simulink model "sampleModel2030"  (R2023a)
settings: Solver=VariableStepAuto  StartTime=0.0  StopTime=10.0  RelTol=1e-3
libraries: hdlsllib x4, simulink x2
settings Model: Creator=user1  LastModifiedBy=user1

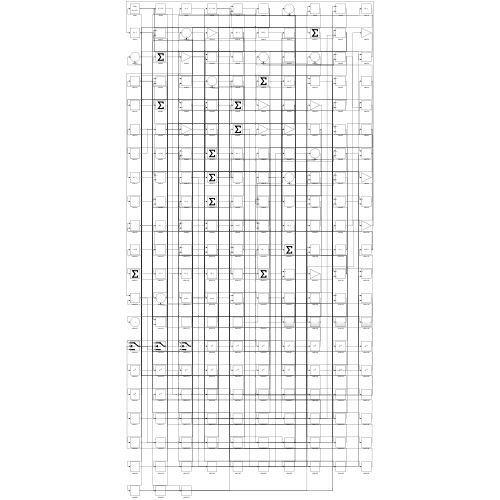
[thumbnail: Simulink's stored preview of the top-level diagram]
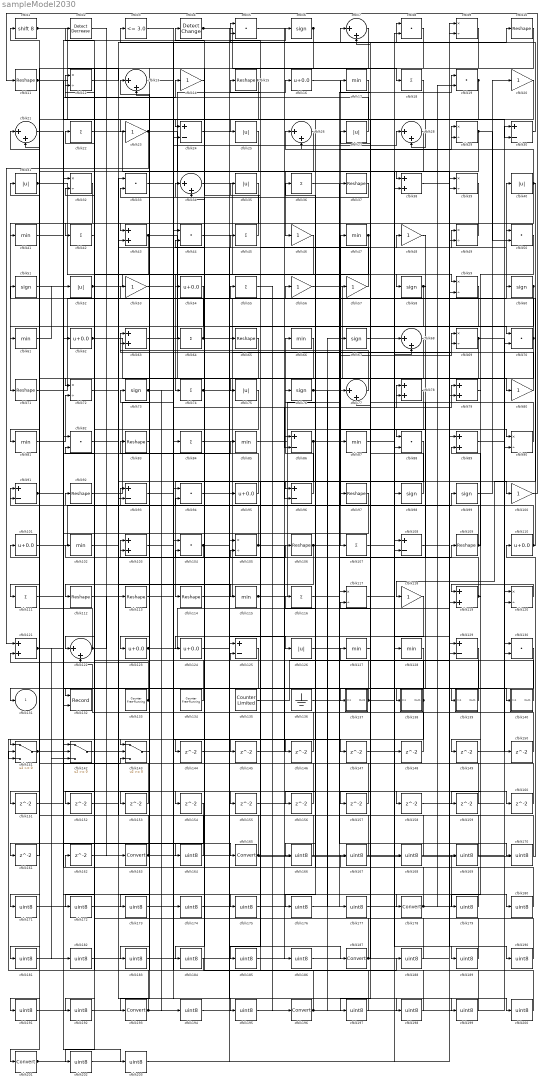
== system sampleModel2030 ==
  cfblk1 : ArithShift  BitShiftNumber=8
  cfblk{10..11,15,37,65,71,83,92,97,106,109,112..114} (14 alike) : Reshape
  cfblk{14,20,23,46,48,53,56..57,80,100,118} (11 alike) : Gain
  cfblk{16,54,62,95,101,110,123..124} (8 alike) : Bias  Bias=0.0  SaturateOnIntegerOverflow=off
  cfblk{17,41,47,61,66,81,85,87,102,115,127..128} (12 alike) : MinMax
  cfblk{38,43,63,78..79,89,103,119,121} (9 alike) : Sum
  cfblk{5,8,19,33,44,50,70,82,88,94,104,130} (12 alike) : DotProduct  OutDataTypeStr=Inherit: Inherit via internal rule
  cfblk{9,12,29,32,39,49,59,69,72,90,105,117,120} (13 alike) : Product  Inputs=*/  RndMeth=Zero  SaturateOnIntegerOverflow=on
  cfblk{18,22,36,42,45,55,64,74,84,107,111,116} (12 alike) : Sum  Inputs=+
  cfblk{24,30,86,91,93,96,108,125,129} (9 alike) : Sum  Inputs=+-
  cfblk{7,13,21,26,28,34,68,77,122} (9 alike) : Sum  Inputs=|++
  cfblk{25,27,31,35,40,52,75,126} (8 alike) : Abs  SaturateOnIntegerOverflow=off
  cfblk132 : Record  FileSettingsInternal="{\"entries\":[{\"content\":{\"excelSettings\":{\"content\":{},\"type\":\"Streamout.ExcelSettings\"}},\"type\":\"Streamout.FileSettingStorage\",\"uuid\":\"\"}],\"packageUris\":[\"http:\\/\\/schema.mathworks.com\\/mf0\\/streamout_blocks\\/R2020a\"],\"version\":\"1.0\"}"  Layout=[1 1]  SignalsInternal="{\"entries\":[{\"content\":{\"signals\":[{\"content\":{\"blockPath\":[],\"dimensions\":[1],\"domain\":\"\",\"lineColor\":\"#a2142f\",\"plots\":[1],\"port\":1,\"signalID\":6116,\"signalName\":\"XY Graph:1\"},\"type\":\"RecordBlkView.Signal\",\"uuid\":\"\"},{\"content\":{\"blockPath\":[],\"dimensions\":[1],\"domain\":\"\",\"lineColor\":\"#139fff\",\"plots\":[1],\"port\":2,\"signalID\":6119,\"signalName\":\"XY Graph:2\"},\"type\":\"RecordBlkView.Signal\",\"uuid\":\"\"}]},\"type\":\"RecordBlkView.InputSignals\",\"uuid\":\"\"}],\"packageUris\":[\"http:\\/\\/schema.mathworks.com\\/mf0\\/streamout_blocks\\/R2020a\"],\"version\":\"1.0\"}"  VisualizationBindings="{\"xyplotplugin\":{\"info\":[{\"series\":[{\"bindingParametersList\":[{\"parameter\":\"X-Axis\",\"signalID\":6116,\"signalName\":\"XY Graph:1\"},{\"parameter\":\"Y-Axis\",\"signalID\":6119,\"signalName\":\"XY Graph:2\"}],\"seriesID\":23883}],\"subplotID\":1}]}}"  CompatibilityTag=XY  st=-1
  cfblk133 : hdlsllib/Sources/Counter Free-Running  NumBits=16  tsamp=-1
  cfblk134 : hdlsllib/Sources/Counter Free-Running  NumBits=16  tsamp=-1
  cfblk135 : hdlsllib/Sources/Counter Limited  uplimit=7  tsamp=-1
  cfblk136 : Ground
  cfblk137 : Subsystem
      settings: LibrarySourceBlock=|
      | hdlsllib/Ports &
      | Subsystems/Subsystem
  cfblk138 : Subsystem
      settings: LibrarySourceBlock=|
      | hdlsllib/Ports &
      | Subsystems/Subsystem
  cfblk139 : Subsystem
      settings: LibrarySourceBlock=|
      | hdlsllib/Ports &
      | Subsystems/Subsystem
  cfblk140 : Subsystem
      settings: LibrarySourceBlock=|
      | hdlsllib/Ports &
      | Subsystems/Subsystem
  cfblk141 : Switch  SaturateOnIntegerOverflow=off  InputSameDT=off
  cfblk142 : Switch  SaturateOnIntegerOverflow=off  InputSameDT=off
  cfblk143 : Switch  SaturateOnIntegerOverflow=off  InputSameDT=off
  cfblk{144..162} (19 alike) : Delay  SampleTime=1
  cfblk{163,165,178,187,193,196,201} (7 alike) : DataTypeConversion  SaturateOnIntegerOverflow=off  RndMeth=Floor
  cfblk{164,166..177,179..186,188..192,194..195,197..200,202..203} (34 alike) : DataTypeConversion  OutDataTypeStr=uint8  SaturateOnIntegerOverflow=off  RndMeth=Floor
  cfblk2 : simulink/Logic and Bit Operations/Detect Decrease  vinit=0.0  OutDataTypeStr=boolean
      settings: LibrarySourceBlock=|
      | hdlsllib/Logic and Bit
      | Operations/Detect
      | Decrease
  cfblk3 : hdlsllib/Logic and Bit Operations/Compare To Constant  relop=<=  const=3.0  OutDataTypeStr=boolean
  cfblk4 : simulink/Logic and Bit Operations/Detect Change  vinit=0  OutDataTypeStr=boolean
      settings: LibrarySourceBlock=|
      | hdlsllib/Logic and Bit
      | Operations/Detect
      | Change
  cfblk{6,51,58,60,67,73,76,98..99} (9 alike) : Signum
  cfblk131 : Outport  VectorParamsAs1DForOutWhenUnconnected=off
  wires:
  cfblk88/1 -> cfblk114/1
  cfblk63/1 -> cfblk16/1
  cfblk99/1 -> cfblk20/1
  cfblk49/1 -> cfblk43/1
  cfblk61/1 -> cfblk52/1
  cfblk122/1 -> cfblk113/1, cfblk91/1
  cfblk134/1 -> cfblk92/1
  cfblk113/1 -> cfblk99/1
  cfblk52/1 -> cfblk58/1, cfblk48/1
  cfblk118/1 -> cfblk143/1
  cfblk71/1 -> cfblk40/1
  cfblk32/1 -> cfblk71/1
  cfblk30/1 -> cfblk5/1
  cfblk16/1 -> cfblk107/1
  cfblk80/1 -> cfblk63/1
  cfblk59/1 -> cfblk137/1(In1)
  cfblk74/1 -> cfblk56/1, cfblk50/1
  cfblk29/1 -> cfblk46/1, cfblk50/2, cfblk26/2
  cfblk114/1 -> cfblk69/1
  cfblk26/1 -> cfblk132/1
  cfblk101/1 -> cfblk47/1
  cfblk106/1 -> cfblk49/1, cfblk192/1
  cfblk137/1(Out1) -> cfblk103/1, cfblk116/1, cfblk29/2
  cfblk31/1 -> cfblk74/1, cfblk175/1
  cfblk56/1 -> cfblk80/1
  cfblk46/1 -> cfblk72/1
  cfblk78/1 -> cfblk87/1
  cfblk97/1 -> cfblk132/2
  cfblk60/1 -> cfblk81/1, cfblk179/1
  cfblk83/1 -> cfblk13/1
  cfblk75/1 -> cfblk112/1
  cfblk77/1 -> cfblk13/2
  cfblk109/1 -> cfblk31/1, cfblk89/2
  cfblk73/1 -> cfblk28/1, cfblk194/1
  cfblk120/1 -> cfblk119/1
  cfblk105/1 -> cfblk34/1, cfblk180/1
  cfblk81/1 -> cfblk72/2
  cfblk55/1 -> cfblk196/1
  cfblk45/1 -> cfblk4/1
  cfblk111/1 -> cfblk62/1
  cfblk44/1 -> cfblk187/1
  cfblk98/1 -> cfblk27/1
  cfblk100/1 -> cfblk11/1
  cfblk23/1 -> cfblk121/1, cfblk89/1, cfblk155/1
  cfblk85/1 -> cfblk90/1
  cfblk43/1 -> cfblk97/1, cfblk143/2
  cfblk10/1 -> cfblk61/1
  cfblk139/1(Out1) -> cfblk57/1
  cfblk136/1 -> cfblk19/1
  cfblk141/1 -> cfblk85/1, cfblk142/3, cfblk143/3
  cfblk37/1 -> cfblk33/2
  cfblk34/1 -> cfblk59/1
  cfblk40/1 -> cfblk118/1, cfblk122/1, cfblk26/1
  cfblk102/1 -> cfblk45/1
  cfblk115/1 -> cfblk77/1, cfblk78/2
  cfblk62/1 -> cfblk120/1, cfblk96/2
  cfblk11/1 -> cfblk25/1, cfblk24/1
  cfblk138/1(Out1) -> cfblk7/1, cfblk141/3
  cfblk35/1 -> cfblk41/1
  cfblk24/1 -> cfblk70/1
  cfblk119/1 -> cfblk102/1, cfblk36/1, cfblk78/1, cfblk159/1
  cfblk124/1 -> cfblk65/1
  cfblk72/1 -> cfblk100/1
  cfblk142/1 -> cfblk106/1
  cfblk64/1 -> cfblk126/1, cfblk12/2
  cfblk33/1 -> cfblk84/1
  cfblk130/1 -> cfblk193/1
  cfblk110/1 -> cfblk77/2, cfblk60/1, cfblk35/1
  cfblk79/1 -> cfblk139/1(In1)
  cfblk69/1 -> cfblk90/2, cfblk111/1
  cfblk58/1 -> cfblk138/1(In1), cfblk166/1
  cfblk121/1 -> cfblk154/1, cfblk182/1
  cfblk39/1 -> cfblk201/1
  cfblk123/1 -> cfblk49/2, cfblk79/1
  cfblk96/1 -> cfblk66/1
  cfblk21/1 -> cfblk165/1
  cfblk92/1 -> cfblk64/1
  cfblk38/1 -> cfblk129/1
  cfblk1/1 -> cfblk30/2, cfblk93/2
  cfblk104/1 -> cfblk103/2, cfblk146/1
  cfblk15/1 -> cfblk141/1, cfblk183/1
  cfblk22/1 -> cfblk98/1
  cfblk6/1 -> cfblk42/1, cfblk23/1, cfblk153/1
  cfblk112/1 -> cfblk115/1
  cfblk91/1 -> cfblk14/1, cfblk140/1(In1)
  cfblk140/1(Out1) -> cfblk127/1
  cfblk51/1 -> cfblk6/1
  cfblk65/1 -> cfblk123/1
  cfblk133/1 -> cfblk121/2, cfblk22/1
  cfblk27/1 -> cfblk12/1
  cfblk76/1 -> cfblk29/1, cfblk177/1
  cfblk95/1 -> cfblk83/1
  cfblk82/1 -> cfblk178/1
  cfblk90/1 -> cfblk3/1
  cfblk129/1 -> cfblk131/1
  cfblk4/1 -> cfblk18/1, cfblk158/1
  cfblk67/1 -> cfblk129/2
  cfblk20/1 -> cfblk54/1
  cfblk70/1 -> cfblk51/1, cfblk164/1
  cfblk2/1 -> cfblk163/1
  cfblk66/1 -> cfblk75/1
  cfblk19/1 -> cfblk43/2, cfblk28/2, cfblk24/2
  cfblk14/1 -> cfblk124/1
  cfblk28/1 -> cfblk38/1
  cfblk53/1 -> cfblk8/1
  cfblk48/1 -> cfblk88/1
  cfblk87/1 -> cfblk38/2
  cfblk47/1 -> cfblk156/1, cfblk172/1
  cfblk5/1 -> cfblk86/2
  cfblk57/1 -> cfblk15/1
  cfblk116/1 -> cfblk109/1
  cfblk143/1 -> cfblk93/1
  cfblk135/1 -> cfblk59/2
  cfblk93/1 -> cfblk96/1
  cfblk86/1 -> cfblk69/2, cfblk185/1
  cfblk12/1 -> cfblk10/1
  cfblk8/1 -> cfblk144/1
  cfblk103/1 -> cfblk145/1
  cfblk145/1 -> cfblk86/1
  cfblk146/1 -> cfblk122/2
  cfblk84/1 -> cfblk147/1
  cfblk107/1 -> cfblk148/1
  cfblk148/1 -> cfblk63/2
  cfblk50/1 -> cfblk149/1
  cfblk149/1 -> cfblk30/1
  cfblk89/1 -> cfblk150/1
  cfblk150/1 -> cfblk34/2
  cfblk25/1 -> cfblk151/1
  cfblk151/1 -> cfblk32/1
  cfblk42/1 -> cfblk152/1
  cfblk153/1 -> cfblk91/2
  cfblk156/1 -> cfblk105/2
  cfblk18/1 -> cfblk157/1
  cfblk157/1 -> cfblk142/2
  cfblk158/1 -> cfblk120/2
  cfblk159/1 -> cfblk5/2
  cfblk36/1 -> cfblk160/1
  cfblk160/1 -> cfblk142/1
  cfblk7/1 -> cfblk161/1
  cfblk161/1 -> cfblk1/1
  cfblk162/1 -> cfblk79/2
  cfblk163/1 -> cfblk88/2, cfblk101/1
  cfblk164/1 -> cfblk2/1
  cfblk165/1 -> cfblk110/1, cfblk104/2, cfblk70/2
  cfblk166/1 -> cfblk21/1
  cfblk167/1 -> cfblk21/2
  cfblk117/1 -> cfblk168/1
  cfblk168/1 -> cfblk33/1
  cfblk169/1 -> cfblk117/1
  cfblk126/1 -> cfblk170/1
  cfblk170/1 -> cfblk117/2
  cfblk128/1 -> cfblk171/1
  cfblk171/1 -> cfblk37/1
  cfblk172/1 -> cfblk128/1
  cfblk125/1 -> cfblk173/1
  cfblk173/1 -> cfblk169/1
  cfblk3/1 -> cfblk174/1
  cfblk174/1 -> cfblk125/1
  cfblk175/1 -> cfblk125/2
  cfblk17/1 -> cfblk176/1
  cfblk176/1 -> cfblk119/2
  cfblk177/1 -> cfblk17/1
  cfblk178/1 -> cfblk76/1, cfblk7/2, cfblk19/2
  cfblk179/1 -> cfblk82/1
  cfblk180/1 -> cfblk82/2
  cfblk68/1 -> cfblk181/1
  cfblk181/1 -> cfblk104/1
  cfblk182/1 -> cfblk68/1
  cfblk183/1 -> cfblk68/2
  cfblk9/1 -> cfblk184/1
  cfblk185/1 -> cfblk9/1
  cfblk155/1 -> cfblk186/1
  cfblk186/1 -> cfblk9/2
  cfblk187/1 -> cfblk167/1, cfblk32/2
  cfblk184/1 -> cfblk188/1
  cfblk188/1 -> cfblk44/1
  cfblk147/1 -> cfblk189/1
  cfblk189/1 -> cfblk44/2
  cfblk108/1 -> cfblk190/1
  cfblk190/1 -> cfblk73/1
  cfblk154/1 -> cfblk191/1
  cfblk191/1 -> cfblk108/1
  cfblk192/1 -> cfblk108/2
  cfblk193/1 -> cfblk162/1, cfblk105/1
  cfblk194/1 -> cfblk130/1
  cfblk152/1 -> cfblk195/1
  cfblk195/1 -> cfblk130/2
  cfblk196/1 -> cfblk141/2, cfblk67/1
  cfblk127/1 -> cfblk197/1
  cfblk197/1 -> cfblk55/1
  cfblk94/1 -> cfblk198/1
  cfblk198/1 -> cfblk53/1
  cfblk144/1 -> cfblk199/1
  cfblk199/1 -> cfblk94/1
  cfblk13/1 -> cfblk200/1
  cfblk200/1 -> cfblk94/2
  cfblk201/1 -> cfblk8/2, cfblk95/1
  cfblk54/1 -> cfblk202/1
  cfblk202/1 -> cfblk39/1
  cfblk41/1 -> cfblk203/1
  cfblk203/1 -> cfblk39/2

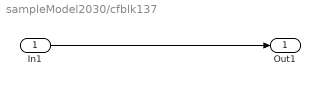
== system sampleModel2030/cfblk137 ==
  In1 : Inport
  Out1 : Outport
  wires:
  In1/1 -> Out1/1

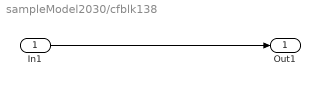
== system sampleModel2030/cfblk138 ==
  In1 : Inport
  Out1 : Outport
  wires:
  In1/1 -> Out1/1

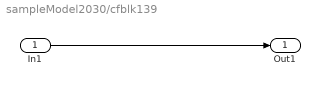
== system sampleModel2030/cfblk139 ==
  In1 : Inport
  Out1 : Outport
  wires:
  In1/1 -> Out1/1

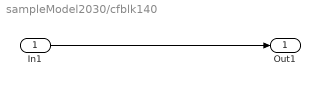
== system sampleModel2030/cfblk140 ==
  In1 : Inport
  Out1 : Outport
  wires:
  In1/1 -> Out1/1
